simulink model "my_PLL_IntegerN_noiseless_3_3"  (R2024b)
settings: Solver=VariableStepAuto  StartTime=0.0  StopTime=1e-3  RelTol=1e-3
model workspace (MAT data in the model file):
  PhaseNoise_42 = [-191.261666509 -181.016259323 -185.62739633]
  PnFrequencyOffset_42 = [50000000 25000000 75000000]
  TargetFrequency_30 = 2100000000
  TargetPhaseNoise_30 = [-85 -125 -150 -180]
  phaseNoiseResultTable = [25000000  -181.016259323  -55; 50000000  -191.261666509  -45; 75000000  -185.62739633  -65]
  resolutionBandwidth = 30000
  uniqueStringPll_30 = '95_7167'
  uniqueString_41 = '91_3376'
  uniqueString_42 = '9_754'
libraries: msbPllFoundation x5
settings Model: VariantFading=off  Creator=BrunoFraga  LastModifiedBy=brunoalexandrefraga

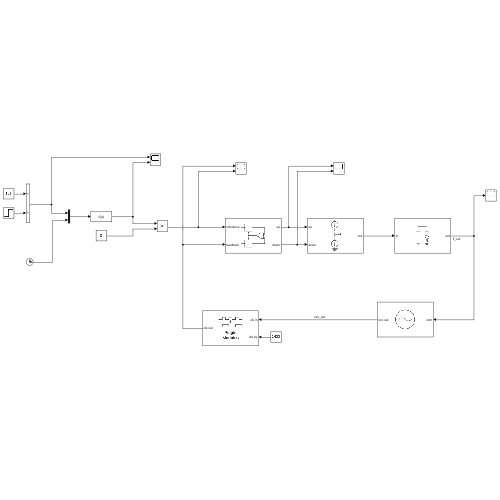
[thumbnail: Simulink's stored preview of the top-level diagram]
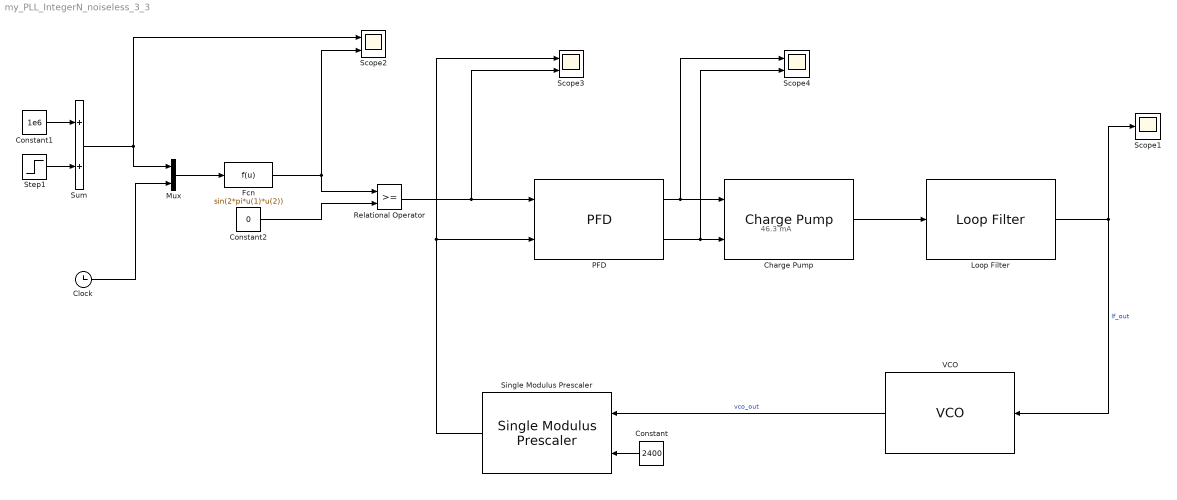
== system my_PLL_IntegerN_noiseless_3_3 ==
  note: 46.3 mA
  Charge Pump : msbPllFoundation/Charge Pump  OutputCurrent=46.3e-6  InputThreshold=1e-18  ExtraBuffer=off  NBuffer=1000  EnableCurrentImpairments=off  CurrentImbalance=1e-4  LeakageCurrent=1e-5  EnableTimingImpairments=off  DefaultOrAdvanced=Default  MaxFreqInterest=10e9  RiseFallUp=50e-12  PropDelayUp=60e-12  RiseFallDown=20e-12  PropDelayDown=40e-12
  Clock : Clock
  Constant : Constant  Value=2400
  Constant1 : Constant  Value=1e6  SampleTime=1e-6
  Constant2 : Constant  Value=0
  Fcn : Fcn  Expr=sin(2*pi*u(1)*u(2))
  Loop Filter : msbPllFoundation/Loop Filter  FilterType=2nd order passive  C1=500e-12  C2=5e-9  C3=1.0452e-15  C4=1e-12  R2=9.09e3  R3=51.0435e6  R4=12e3  ExtraBuffer=off  NBuffer=1000  EnableImpairments=off  Temperature=30
  Mux : Mux  Inputs=2
  PFD : msbPllFoundation/PFD  DeadbandCompensation=30e-12  ExtraBuffer=off  NBuffer=1000  EnableImpairments=off  DefaultOrAdvanced=Default  MaxFreqInterest=10e9  RiseFallTime=30e-12  PropDelay=50e-12
  Relational Operator : RelationalOperator  OutDataTypeStr=boolean  RndMeth=Simplest  InputSameDT=off
  Scope1 : Scope
  Scope2 : Scope  NumInputPorts=2
  Scope3 : Scope  NumInputPorts=2
  Scope4 : Scope  NumInputPorts=2
  Single Modulus Prescaler : msbPllFoundation/Single Modulus Prescaler  ExtraBuffer=off  NBuffer=1000
  Step1 : Step  Time=350e-6  After=65e3  SampleTime=200e-6
  Sum : Sum
  VCO : msbPllFoundation/VCO  SpecifyUsing=Voltage sensitivity  Kvco=250e6  Fo=2.19175e9  ControlVoltage=[-5 0 10]  OutputFrequency=[100 50e6 150e6]  Amplitude=1  ExtraBuffer=off  NBuffer=1000  AddPhaseNoise=off  Foffset=[10e3 100e3 1e6 3e6 10e6]  PhaseNoise=[-77 -108 -134 -145 -154]  MaxKvco=250000000
  wires:
  Relational Operator/1 -> Scope3/2, PFD/1
  VCO/1 -> Single Modulus Prescaler/1  "vco_out"
  Constant/1 -> Single Modulus Prescaler/2
  Charge Pump/1 -> Loop Filter/1
  PFD/1 -> Scope4/1, Charge Pump/1
  Single Modulus Prescaler/1 -> Scope3/1, PFD/2
  Loop Filter/1 -> VCO/1, Scope1/1  "lf_out"
  PFD/2 -> Scope4/2, Charge Pump/2
  Constant2/1 -> Relational Operator/2
  Fcn/1 -> Scope2/2, Relational Operator/1
  Constant1/1 -> Sum/1
  Mux/1 -> Fcn/1
  Clock/1 -> Mux/2
  Sum/1 -> Mux/1, Scope2/1
  Step1/1 -> Sum/2
